simulink model "ksrbl_4k4t_hdtrig"  (Simulink 6.2)
settings: Solver=ode45  StartTime=0.0  StopTime=20000  RelTol=1e-3
libraries: xbsIndex_r3 x1214, casper_library x120, xps_library x20
(part 13 of 26)

== system ksrbl_4k4t_hdtrig/pfb_fir_real/pol1_in2_last_tap/pfb_real_add_tree ==
  din : Inport  Port=1  LatchInput=off
  sync : Inport  Port=2  LatchInput=off
  Reint{0..3} (4 alike) : xbsIndex_r3/Reinterpret  force_arith_type=on  arith_type="Signed  (2's comp)"  force_bin_pt=on  bin_pt=CoeffBitWidth + BitWidthIn - 2  force_valid=on
  Slice0 : xbsIndex_r3/Slice  mode=Upper Bit Location + Width  nbits=CoeffBitWidth + BitWidthIn  bit1=-0*(CoeffBitWidth + BitWidthIn)  base1=MSB of Input  bit0=0  base0=MSB of Input  boolean_output=off  explicit_period=off  period=1  dbl_ovrd=off
  Slice1 : xbsIndex_r3/Slice  mode=Upper Bit Location + Width  nbits=CoeffBitWidth + BitWidthIn  bit1=-1*(CoeffBitWidth + BitWidthIn)  base1=MSB of Input  bit0=0  base0=MSB of Input  boolean_output=off  explicit_period=off  period=1  dbl_ovrd=off
  Slice2 : xbsIndex_r3/Slice  mode=Upper Bit Location + Width  nbits=CoeffBitWidth + BitWidthIn  bit1=-2*(CoeffBitWidth + BitWidthIn)  base1=MSB of Input  bit0=0  base0=MSB of Input  boolean_output=off  explicit_period=off  period=1  dbl_ovrd=off
  Slice3 : xbsIndex_r3/Slice  mode=Upper Bit Location + Width  nbits=CoeffBitWidth + BitWidthIn  bit1=-3*(CoeffBitWidth + BitWidthIn)  base1=MSB of Input  bit0=0  base0=MSB of Input  boolean_output=off  explicit_period=off  period=1  dbl_ovrd=off
  adder_tree1 : Subsystem  AncestorBlock=casper_library/Misc/adder_tree  mask(adder_tree){n_inputs=4, latency=4}
      mask prompts: n_inputs "Number of Inputs"; latency "Add Latency"
      mask help: Sums all inputs using a tree of adds and delays.
      mask init:
      | adder_tree_init(gcb, ...
      |     'n_inputs', n_inputs, ...
      |     'latency', latency);
      settings: AttributesFormatString=latency 8
      mask Help: eval('xlWeb([getenv(''MLIB_ROOT''), ''\doc\html\sp_adder_tree\sp_adder_tree.html''])')
  convert1 : xbsIndex_r3/Convert  arith_type="Signed  (2's comp)"  n_bits=BitWidthOut  bin_pt=BitWidthOut-1  quantization=Truncate  overflow=Saturate  latency=add_latency  explicit_period=off  period=1  dbl_ovrd=off  show_param=off  inserted_by_tool=off  pipeline=off
      settings: xl_area=[0, 0, 0, 0, 0, 0, 0]
  delay1 : xbsIndex_r3/Delay  latency=4  reg_retiming=off  explicit_period=off  period=1  en=off  accept_only_valid=off  init_zero=on  dbl_ovrd=off  show_param=off
      settings: xl_area=[0, 0, 0, 0, 0, 0, 0]
  scale1 : xbsIndex_r3/Scale  scale_factor=-3  explicit_period=off  period=1  dbl_ovrd=off
  dout : Outport
  sync_out : Outport  Port=2
  wires:
  adder_tree1/2(dout) -> scale1/1
  scale1/1 -> convert1/1
  convert1/1 -> dout/1
  sync/1 -> adder_tree1/1(sync)
  adder_tree1/1(sync_out) -> delay1/1
  delay1/1 -> sync_out/1
  din/1 -> Slice0/1, Slice1/1, Slice2/1, Slice3/1
  Slice0/1 -> Reint0/1
  Reint0/1 -> adder_tree1/2(din1)
  Slice1/1 -> Reint1/1
  Reint1/1 -> adder_tree1/3(din2)
  Slice2/1 -> Reint2/1
  Reint2/1 -> adder_tree1/4(din3)
  Slice3/1 -> Reint3/1
  Reint3/1 -> adder_tree1/5(din4)

== system ksrbl_4k4t_hdtrig/pfb_fir_real/pol1_in3_first_tap/delay ==
  In1 : Inport  Port=1  LatchInput=off
  delay_bram : casper_library/Delays/delay_bram  DelayLen=2^(PFBSize-n_inputs)  bram_latency=bram_latency
  Out1 : Outport
  wires:
  In1/1 -> delay_bram/1
  delay_bram/1 -> Out1/1
